simulink model "SVPWM"  (R2018b)
settings: Solver=FixedStepAuto  StartTime=0.0  StopTime=0.1  RelTol=1e-3
undefined symbols (not defined in the file): gcbh, Newton, Raphson, sps_rtmsupport
libraries: powerlib x60, powerlib_meascontrol x25, simulink x14, dspstat3 x1
(part 2 of 2)

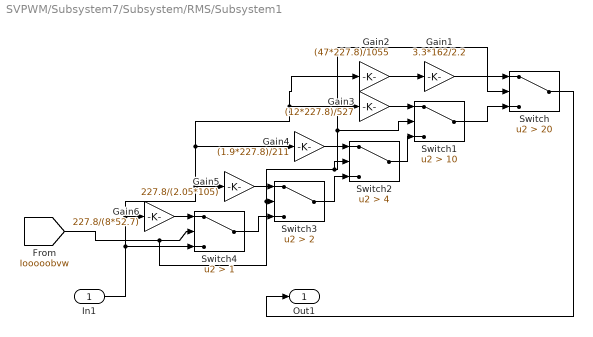
== system SVPWM/Subsystem7/Subsystem/RMS/Subsystem1 ==
  In1 : Inport
  Gain1 : Gain  Gain=3.3*162/2.2
  Gain2 : Gain  Gain=(47*227.8)/1055
  Gain3 : Gain  Gain=(12*227.8)/527
  Gain4 : Gain  Gain=(1.9*227.8)/211
  Gain5 : Gain  Gain=227.8/(2.05*105)
  Gain6 : Gain  Gain=227.8/(8*52.7)
  Switch : Switch  Criteria=u2 > Threshold  Threshold=20
  Switch1 : Switch  Criteria=u2 > Threshold  Threshold=10
  Switch2 : Switch  Criteria=u2 > Threshold  Threshold=4
  Switch3 : Switch  Criteria=u2 > Threshold  Threshold=2
  Switch4 : Switch  Criteria=u2 > Threshold  Threshold=1
  Out1 : Outport
  wires:
  Gain1/1 -> Switch/1
  Switch/1 -> Out1/1
  Gain6/1 -> Switch4/1
  Switch4/1 -> Switch3/3
  Switch2/1 -> Switch1/3
  Gain2/1 -> Gain1/1
  Gain5/1 -> Switch3/1
  Gain4/1 -> Switch2/1
  Switch3/1 -> Switch2/3
  Gain3/1 -> Switch1/1
  [Iooooobvw] -> Switch4/2, Switch3/2, Switch2/2, Switch1/2, Switch/2
  In1/1 -> Gain2/1, Gain3/1, Gain4/1, Gain5/1, Gain6/1, Switch4/3
  Switch1/1 -> Switch/3

== system SVPWM/Subsystem7/Subsystem/RMS/TrueRMS  ==
  In : Inport
  Enable : EnablePort
  Mean value : powerlib_meascontrol/Measurements/Mean  Freq=sps.Freq  Vinit=sps.Par_Init_TrueRMS  Ts=Ts
  Product : Product  SaturateOnIntegerOverflow=on  InputSameDT=on  OutDataTypeStr=Inherit: Same as first input
  Saturation to avoid negative sqrt : Saturate  UpperLimit=Inf  LowerLimit=0
  Sqrt : Sqrt  AlgorithmType=Newton-Raphson  SaturateOnIntegerOverflow=on
  RMS : Outport
  wires:
  Saturation to avoid negative sqrt/1 -> Sqrt/1
  Mean value/1 -> Saturation to avoid negative sqrt/1
  Product/1 -> Mean value/1
  In/1 -> Product/2, Product/1
  Sqrt/1 -> RMS/1

== system SVPWM/Subsystem7/Subsystem/Subsystem/Subsystem ==
  In1 : Inport
  In2 : Inport  Port=2
  Demux : Demux  Outputs=6
  Logical Operator : Logic  IconShape=distinctive  AllPortsSameDT=off  OutDataTypeStr=boolean
  Scope : Scope  NumInputPorts=2
  Switch : Switch  Criteria=u2 > Threshold
  Out1 : Outport
  wires:
  Demux/2 -> Scope/1, Switch/3
  Switch/1 -> Logical Operator/2
  [svpwm] -> Demux/1
  Logical Operator/1 -> Out1/1
  In1/1 -> Scope/2, Logical Operator/1
  In2/1 -> Switch/2

== system SVPWM/Subsystem7/Subsystem/Subsystem/Subsystem1 ==
  In1 : Inport
  In2 : Inport  Port=2
  Demux : Demux  Outputs=6
  Logical Operator : Logic  IconShape=distinctive  AllPortsSameDT=off  OutDataTypeStr=boolean
  SVPWM Generator (2-Level) : powerlib_meascontrol/Pulse & Signal Generators/SVPWM Generator (2-Level)  InputType=Internally generated  SwitchingPattern=Pattern #2  Fc=100  ParUref=[1 -60 50]  Ts=0
      settings: SourceProductName=Simscape Power Systems  SourceProductBaseCode=PS
  Scope : Scope  NumInputPorts=2
  Switch : Switch  Criteria=u2 > Threshold
  Out1 : Outport
  tag scope: svpwm=global
  wires:
  In2/1 -> Switch/2
  In1/1 -> Scope/2, Logical Operator/1
  Logical Operator/1 -> Out1/1
  SVPWM Generator (2-Level)/1 -> [svpwm], Demux/1
  Switch/1 -> Logical Operator/2
  Demux/1 -> Scope/1, Switch/1

== system SVPWM/Subsystem7/Subsystem1/RMS/RMS  ==
  In : Inport
  Enable : EnablePort
  Fourier1 : powerlib_meascontrol/Measurements/Fourier  Freq=sps.Freq  n=1  InInit=sps.Par_Init_RMS  Ts=Ts
      settings: SourceProductName=Simscape Power Systems
  Gain : Gain  Gain=1/sqrt(2)
  Terminator : Terminator
  RMS : Outport
  wires:
  Fourier1/1 -> Gain/1
  Fourier1/2 -> Terminator/1
  In/1 -> Fourier1/1
  Gain/1 -> RMS/1

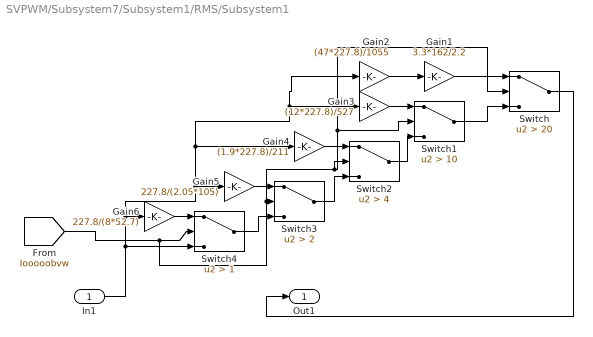
== system SVPWM/Subsystem7/Subsystem1/RMS/Subsystem1 ==
  In1 : Inport
  Gain1 : Gain  Gain=3.3*162/2.2
  Gain2 : Gain  Gain=(47*227.8)/1055
  Gain3 : Gain  Gain=(12*227.8)/527
  Gain4 : Gain  Gain=(1.9*227.8)/211
  Gain5 : Gain  Gain=227.8/(2.05*105)
  Gain6 : Gain  Gain=227.8/(8*52.7)
  Switch : Switch  Criteria=u2 > Threshold  Threshold=20
  Switch1 : Switch  Criteria=u2 > Threshold  Threshold=10
  Switch2 : Switch  Criteria=u2 > Threshold  Threshold=4
  Switch3 : Switch  Criteria=u2 > Threshold  Threshold=2
  Switch4 : Switch  Criteria=u2 > Threshold  Threshold=1
  Out1 : Outport
  wires:
  Gain1/1 -> Switch/1
  Switch/1 -> Out1/1
  Gain6/1 -> Switch4/1
  Switch4/1 -> Switch3/3
  Switch2/1 -> Switch1/3
  Gain2/1 -> Gain1/1
  Gain5/1 -> Switch3/1
  Gain4/1 -> Switch2/1
  Switch3/1 -> Switch2/3
  Gain3/1 -> Switch1/1
  [Iooooobvw] -> Switch4/2, Switch3/2, Switch2/2, Switch1/2, Switch/2
  In1/1 -> Gain2/1, Gain3/1, Gain4/1, Gain5/1, Gain6/1, Switch4/3
  Switch1/1 -> Switch/3

== system SVPWM/Subsystem7/Subsystem1/RMS/TrueRMS  ==
  In : Inport
  Enable : EnablePort
  Mean value : powerlib_meascontrol/Measurements/Mean  Freq=sps.Freq  Vinit=sps.Par_Init_TrueRMS  Ts=Ts
  Product : Product  SaturateOnIntegerOverflow=on  InputSameDT=on  OutDataTypeStr=Inherit: Same as first input
  Saturation to avoid negative sqrt : Saturate  UpperLimit=Inf  LowerLimit=0
  Sqrt : Sqrt  AlgorithmType=Newton-Raphson  SaturateOnIntegerOverflow=on
  RMS : Outport
  wires:
  Saturation to avoid negative sqrt/1 -> Sqrt/1
  Mean value/1 -> Saturation to avoid negative sqrt/1
  Product/1 -> Mean value/1
  In/1 -> Product/2, Product/1
  Sqrt/1 -> RMS/1

== system SVPWM/Subsystem7/Subsystem1/Subsystem7/Subsystem ==
  In1 : Inport
  In2 : Inport  Port=2
  Demux : Demux  Outputs=6
  Logical Operator : Logic  IconShape=distinctive  AllPortsSameDT=off  OutDataTypeStr=boolean
  Scope : Scope  NumInputPorts=2
  Switch : Switch  Criteria=u2 > Threshold
  Out1 : Outport
  wires:
  Demux/2 -> Scope/1, Switch/3
  Switch/1 -> Logical Operator/2
  [svpwm] -> Demux/1
  Logical Operator/1 -> Out1/1
  In1/1 -> Scope/2, Logical Operator/1
  In2/1 -> Switch/2

== system SVPWM/Subsystem7/Subsystem1/Subsystem7/Subsystem1 ==
  In1 : Inport
  In2 : Inport  Port=2
  Demux : Demux  Outputs=6
  Logical Operator : Logic  IconShape=distinctive  AllPortsSameDT=off  OutDataTypeStr=boolean
  Scope : Scope  NumInputPorts=2
  Switch : Switch  Criteria=u2 > Threshold
  Out1 : Outport
  wires:
  In2/1 -> Switch/2
  In1/1 -> Scope/2, Logical Operator/1
  Logical Operator/1 -> Out1/1
  [svpwm] -> Demux/1
  Switch/1 -> Logical Operator/2
  Demux/1 -> Scope/1, Switch/1

== system SVPWM/Subsystem7/Subsystem2/RMS/RMS  ==
  In : Inport
  Enable : EnablePort
  Fourier1 : powerlib_meascontrol/Measurements/Fourier  Freq=sps.Freq  n=1  InInit=sps.Par_Init_RMS  Ts=Ts
      settings: SourceProductName=Simscape Power Systems
  Gain : Gain  Gain=1/sqrt(2)
  Terminator : Terminator
  RMS : Outport
  wires:
  Fourier1/1 -> Gain/1
  Fourier1/2 -> Terminator/1
  In/1 -> Fourier1/1
  Gain/1 -> RMS/1

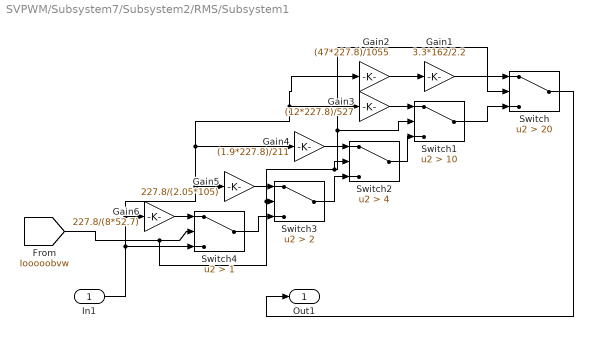
== system SVPWM/Subsystem7/Subsystem2/RMS/Subsystem1 ==
  In1 : Inport
  Gain1 : Gain  Gain=3.3*162/2.2
  Gain2 : Gain  Gain=(47*227.8)/1055
  Gain3 : Gain  Gain=(12*227.8)/527
  Gain4 : Gain  Gain=(1.9*227.8)/211
  Gain5 : Gain  Gain=227.8/(2.05*105)
  Gain6 : Gain  Gain=227.8/(8*52.7)
  Switch : Switch  Criteria=u2 > Threshold  Threshold=20
  Switch1 : Switch  Criteria=u2 > Threshold  Threshold=10
  Switch2 : Switch  Criteria=u2 > Threshold  Threshold=4
  Switch3 : Switch  Criteria=u2 > Threshold  Threshold=2
  Switch4 : Switch  Criteria=u2 > Threshold  Threshold=1
  Out1 : Outport
  wires:
  Gain1/1 -> Switch/1
  Switch/1 -> Out1/1
  Gain6/1 -> Switch4/1
  Switch4/1 -> Switch3/3
  Switch2/1 -> Switch1/3
  Gain2/1 -> Gain1/1
  Gain5/1 -> Switch3/1
  Gain4/1 -> Switch2/1
  Switch3/1 -> Switch2/3
  Gain3/1 -> Switch1/1
  [Iooooobvw] -> Switch4/2, Switch3/2, Switch2/2, Switch1/2, Switch/2
  In1/1 -> Gain2/1, Gain3/1, Gain4/1, Gain5/1, Gain6/1, Switch4/3
  Switch1/1 -> Switch/3

== system SVPWM/Subsystem7/Subsystem2/RMS/TrueRMS  ==
  In : Inport
  Enable : EnablePort
  Mean value : powerlib_meascontrol/Measurements/Mean  Freq=sps.Freq  Vinit=sps.Par_Init_TrueRMS  Ts=Ts
  Product : Product  SaturateOnIntegerOverflow=on  InputSameDT=on  OutDataTypeStr=Inherit: Same as first input
  Saturation to avoid negative sqrt : Saturate  UpperLimit=Inf  LowerLimit=0
  Sqrt : Sqrt  AlgorithmType=Newton-Raphson  SaturateOnIntegerOverflow=on
  RMS : Outport
  wires:
  Saturation to avoid negative sqrt/1 -> Sqrt/1
  Mean value/1 -> Saturation to avoid negative sqrt/1
  Product/1 -> Mean value/1
  In/1 -> Product/2, Product/1
  Sqrt/1 -> RMS/1

== system SVPWM/Subsystem7/Subsystem2/Subsystem/Subsystem ==
  In1 : Inport
  In2 : Inport  Port=2
  Demux : Demux  Outputs=6
  Logical Operator : Logic  IconShape=distinctive  AllPortsSameDT=off  OutDataTypeStr=boolean
  Scope : Scope  NumInputPorts=2
  Switch : Switch  Criteria=u2 > Threshold
  Out1 : Outport
  wires:
  Demux/2 -> Scope/1, Switch/3
  Switch/1 -> Logical Operator/2
  [svpwm] -> Demux/1
  Logical Operator/1 -> Out1/1
  In1/1 -> Scope/2, Logical Operator/1
  In2/1 -> Switch/2

== system SVPWM/Subsystem7/Subsystem2/Subsystem/Subsystem1 ==
  In1 : Inport
  In2 : Inport  Port=2
  Demux : Demux  Outputs=6
  Logical Operator : Logic  IconShape=distinctive  AllPortsSameDT=off  OutDataTypeStr=boolean
  Scope : Scope  NumInputPorts=2
  Switch : Switch  Criteria=u2 > Threshold
  Out1 : Outport
  wires:
  In2/1 -> Switch/2
  In1/1 -> Scope/2, Logical Operator/1
  Logical Operator/1 -> Out1/1
  [svpwm] -> Demux/1
  Switch/1 -> Logical Operator/2
  Demux/1 -> Scope/1, Switch/1

== system SVPWM/Subsystem7/Subsystem3/RMS/RMS  ==
  In : Inport
  Enable : EnablePort
  Fourier1 : powerlib_meascontrol/Measurements/Fourier  Freq=sps.Freq  n=1  InInit=sps.Par_Init_RMS  Ts=Ts
      settings: SourceProductName=Simscape Power Systems
  Gain : Gain  Gain=1/sqrt(2)
  Terminator : Terminator
  RMS : Outport
  wires:
  Fourier1/1 -> Gain/1
  Fourier1/2 -> Terminator/1
  In/1 -> Fourier1/1
  Gain/1 -> RMS/1

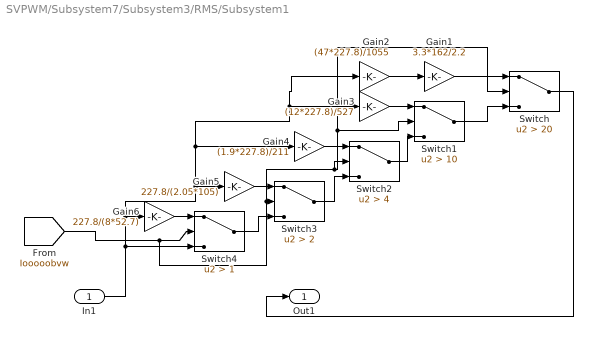
== system SVPWM/Subsystem7/Subsystem3/RMS/Subsystem1 ==
  In1 : Inport
  Gain1 : Gain  Gain=3.3*162/2.2
  Gain2 : Gain  Gain=(47*227.8)/1055
  Gain3 : Gain  Gain=(12*227.8)/527
  Gain4 : Gain  Gain=(1.9*227.8)/211
  Gain5 : Gain  Gain=227.8/(2.05*105)
  Gain6 : Gain  Gain=227.8/(8*52.7)
  Switch : Switch  Criteria=u2 > Threshold  Threshold=20
  Switch1 : Switch  Criteria=u2 > Threshold  Threshold=10
  Switch2 : Switch  Criteria=u2 > Threshold  Threshold=4
  Switch3 : Switch  Criteria=u2 > Threshold  Threshold=2
  Switch4 : Switch  Criteria=u2 > Threshold  Threshold=1
  Out1 : Outport
  wires:
  Gain1/1 -> Switch/1
  Switch/1 -> Out1/1
  Gain6/1 -> Switch4/1
  Switch4/1 -> Switch3/3
  Switch2/1 -> Switch1/3
  Gain2/1 -> Gain1/1
  Gain5/1 -> Switch3/1
  Gain4/1 -> Switch2/1
  Switch3/1 -> Switch2/3
  Gain3/1 -> Switch1/1
  [Iooooobvw] -> Switch4/2, Switch3/2, Switch2/2, Switch1/2, Switch/2
  In1/1 -> Gain2/1, Gain3/1, Gain4/1, Gain5/1, Gain6/1, Switch4/3
  Switch1/1 -> Switch/3

== system SVPWM/Subsystem7/Subsystem3/RMS/TrueRMS  ==
  In : Inport
  Enable : EnablePort
  Mean value : powerlib_meascontrol/Measurements/Mean  Freq=sps.Freq  Vinit=sps.Par_Init_TrueRMS  Ts=Ts
  Product : Product  SaturateOnIntegerOverflow=on  InputSameDT=on  OutDataTypeStr=Inherit: Same as first input
  Saturation to avoid negative sqrt : Saturate  UpperLimit=Inf  LowerLimit=0
  Sqrt : Sqrt  AlgorithmType=Newton-Raphson  SaturateOnIntegerOverflow=on
  RMS : Outport
  wires:
  Saturation to avoid negative sqrt/1 -> Sqrt/1
  Mean value/1 -> Saturation to avoid negative sqrt/1
  Product/1 -> Mean value/1
  In/1 -> Product/2, Product/1
  Sqrt/1 -> RMS/1

== system SVPWM/Subsystem7/Subsystem3/Subsystem/Subsystem ==
  In1 : Inport
  In2 : Inport  Port=2
  Demux : Demux  Outputs=6
  Logical Operator : Logic  IconShape=distinctive  AllPortsSameDT=off  OutDataTypeStr=boolean
  Scope : Scope  NumInputPorts=2
  Switch : Switch  Criteria=u2 > Threshold
  Out1 : Outport
  wires:
  Demux/2 -> Scope/1, Switch/3
  Switch/1 -> Logical Operator/2
  [svpwm] -> Demux/1
  Logical Operator/1 -> Out1/1
  In1/1 -> Scope/2, Logical Operator/1
  In2/1 -> Switch/2

== system SVPWM/Subsystem7/Subsystem3/Subsystem/Subsystem1 ==
  In1 : Inport
  In2 : Inport  Port=2
  Demux : Demux  Outputs=6
  Logical Operator : Logic  IconShape=distinctive  AllPortsSameDT=off  OutDataTypeStr=boolean
  Scope : Scope  NumInputPorts=2
  Switch : Switch  Criteria=u2 > Threshold
  Out1 : Outport
  wires:
  In2/1 -> Switch/2
  In1/1 -> Scope/2, Logical Operator/1
  Logical Operator/1 -> Out1/1
  [svpwm] -> Demux/1
  Switch/1 -> Logical Operator/2
  Demux/1 -> Scope/1, Switch/1

== system SVPWM/Subsystem7/Subsystem4/RMS/RMS  ==
  In : Inport
  Enable : EnablePort
  Fourier1 : powerlib_meascontrol/Measurements/Fourier  Freq=sps.Freq  n=1  InInit=sps.Par_Init_RMS  Ts=Ts
      settings: SourceProductName=Simscape Power Systems
  Gain : Gain  Gain=1/sqrt(2)
  Terminator : Terminator
  RMS : Outport
  wires:
  Fourier1/1 -> Gain/1
  Fourier1/2 -> Terminator/1
  In/1 -> Fourier1/1
  Gain/1 -> RMS/1

== system SVPWM/Subsystem7/Subsystem4/RMS/Subsystem1 ==
  In1 : Inport
  Gain1 : Gain  Gain=3.3*162/2.2
  Gain2 : Gain  Gain=(47*227.8)/1055
  Gain3 : Gain  Gain=(12*227.8)/527
  Gain4 : Gain  Gain=(1.9*227.8)/211
  Gain5 : Gain  Gain=227.8/(2.05*105)
  Gain6 : Gain  Gain=227.8/(8*52.7)
  Switch : Switch  Criteria=u2 > Threshold  Threshold=20
  Switch1 : Switch  Criteria=u2 > Threshold  Threshold=10
  Switch2 : Switch  Criteria=u2 > Threshold  Threshold=4
  Switch3 : Switch  Criteria=u2 > Threshold  Threshold=2
  Switch4 : Switch  Criteria=u2 > Threshold  Threshold=1
  Out1 : Outport
  wires:
  Gain1/1 -> Switch/1
  Switch/1 -> Out1/1
  Gain6/1 -> Switch4/1
  Switch4/1 -> Switch3/3
  Switch2/1 -> Switch1/3
  Gain2/1 -> Gain1/1
  Gain5/1 -> Switch3/1
  Gain4/1 -> Switch2/1
  Switch3/1 -> Switch2/3
  Gain3/1 -> Switch1/1
  [Iooooobvw] -> Switch4/2, Switch3/2, Switch2/2, Switch1/2, Switch/2
  In1/1 -> Gain2/1, Gain3/1, Gain4/1, Gain5/1, Gain6/1, Switch4/3
  Switch1/1 -> Switch/3

== system SVPWM/Subsystem7/Subsystem4/RMS/TrueRMS  ==
  In : Inport
  Enable : EnablePort
  Mean value : powerlib_meascontrol/Measurements/Mean  Freq=sps.Freq  Vinit=sps.Par_Init_TrueRMS  Ts=Ts
  Product : Product  SaturateOnIntegerOverflow=on  InputSameDT=on  OutDataTypeStr=Inherit: Same as first input
  Saturation to avoid negative sqrt : Saturate  UpperLimit=Inf  LowerLimit=0
  Sqrt : Sqrt  AlgorithmType=Newton-Raphson  SaturateOnIntegerOverflow=on
  RMS : Outport
  wires:
  Saturation to avoid negative sqrt/1 -> Sqrt/1
  Mean value/1 -> Saturation to avoid negative sqrt/1
  Product/1 -> Mean value/1
  In/1 -> Product/2, Product/1
  Sqrt/1 -> RMS/1

== system SVPWM/Subsystem7/Subsystem4/Subsystem/Subsystem ==
  In1 : Inport
  In2 : Inport  Port=2
  Demux : Demux  Outputs=6
  Logical Operator : Logic  IconShape=distinctive  AllPortsSameDT=off  OutDataTypeStr=boolean
  Scope : Scope  NumInputPorts=2
  Switch : Switch  Criteria=u2 > Threshold
  Out1 : Outport
  wires:
  Demux/2 -> Scope/1, Switch/3
  Switch/1 -> Logical Operator/2
  [svpwm] -> Demux/1
  Logical Operator/1 -> Out1/1
  In1/1 -> Scope/2, Logical Operator/1
  In2/1 -> Switch/2

== system SVPWM/Subsystem7/Subsystem4/Subsystem/Subsystem1 ==
  In1 : Inport
  In2 : Inport  Port=2
  Demux : Demux  Outputs=6
  Logical Operator : Logic  IconShape=distinctive  AllPortsSameDT=off  OutDataTypeStr=boolean
  Scope : Scope  NumInputPorts=2
  Switch : Switch  Criteria=u2 > Threshold
  Out1 : Outport
  wires:
  In2/1 -> Switch/2
  In1/1 -> Scope/2, Logical Operator/1
  Logical Operator/1 -> Out1/1
  [svpwm] -> Demux/1
  Switch/1 -> Logical Operator/2
  Demux/1 -> Scope/1, Switch/1

== system SVPWM/Subsystem7/Subsystem5/RMS/RMS  ==
  In : Inport
  Enable : EnablePort
  Fourier1 : powerlib_meascontrol/Measurements/Fourier  Freq=sps.Freq  n=1  InInit=sps.Par_Init_RMS  Ts=Ts
      settings: SourceProductName=Simscape Power Systems
  Gain : Gain  Gain=1/sqrt(2)
  Terminator : Terminator
  RMS : Outport
  wires:
  Fourier1/1 -> Gain/1
  Fourier1/2 -> Terminator/1
  In/1 -> Fourier1/1
  Gain/1 -> RMS/1

== system SVPWM/Subsystem7/Subsystem5/RMS/Subsystem1 ==
  In1 : Inport
  Gain1 : Gain  Gain=3.3*162/2.2
  Gain2 : Gain  Gain=(47*227.8)/1055
  Gain3 : Gain  Gain=(12*227.8)/527
  Gain4 : Gain  Gain=(1.9*227.8)/211
  Gain5 : Gain  Gain=227.8/(2.05*105)
  Gain6 : Gain  Gain=227.8/(8*52.7)
  Switch : Switch  Criteria=u2 > Threshold  Threshold=20
  Switch1 : Switch  Criteria=u2 > Threshold  Threshold=10
  Switch2 : Switch  Criteria=u2 > Threshold  Threshold=4
  Switch3 : Switch  Criteria=u2 > Threshold  Threshold=2
  Switch4 : Switch  Criteria=u2 > Threshold  Threshold=1
  Out1 : Outport
  wires:
  Gain1/1 -> Switch/1
  Switch/1 -> Out1/1
  Gain6/1 -> Switch4/1
  Switch4/1 -> Switch3/3
  Switch2/1 -> Switch1/3
  Gain2/1 -> Gain1/1
  Gain5/1 -> Switch3/1
  Gain4/1 -> Switch2/1
  Switch3/1 -> Switch2/3
  Gain3/1 -> Switch1/1
  [Iooooobvw] -> Switch4/2, Switch3/2, Switch2/2, Switch1/2, Switch/2
  In1/1 -> Gain2/1, Gain3/1, Gain4/1, Gain5/1, Gain6/1, Switch4/3
  Switch1/1 -> Switch/3

== system SVPWM/Subsystem7/Subsystem5/RMS/TrueRMS  ==
  In : Inport
  Enable : EnablePort
  Mean value : powerlib_meascontrol/Measurements/Mean  Freq=sps.Freq  Vinit=sps.Par_Init_TrueRMS  Ts=Ts
  Product : Product  SaturateOnIntegerOverflow=on  InputSameDT=on  OutDataTypeStr=Inherit: Same as first input
  Saturation to avoid negative sqrt : Saturate  UpperLimit=Inf  LowerLimit=0
  Sqrt : Sqrt  AlgorithmType=Newton-Raphson  SaturateOnIntegerOverflow=on
  RMS : Outport
  wires:
  Saturation to avoid negative sqrt/1 -> Sqrt/1
  Mean value/1 -> Saturation to avoid negative sqrt/1
  Product/1 -> Mean value/1
  In/1 -> Product/2, Product/1
  Sqrt/1 -> RMS/1

== system SVPWM/Subsystem7/Subsystem5/Subsystem/Subsystem ==
  In1 : Inport
  In2 : Inport  Port=2
  Demux : Demux  Outputs=6
  Logical Operator : Logic  IconShape=distinctive  AllPortsSameDT=off  OutDataTypeStr=boolean
  Scope : Scope  NumInputPorts=2
  Switch : Switch  Criteria=u2 > Threshold
  Out1 : Outport
  wires:
  Demux/2 -> Scope/1, Switch/3
  Switch/1 -> Logical Operator/2
  [svpwm] -> Demux/1
  Logical Operator/1 -> Out1/1
  In1/1 -> Scope/2, Logical Operator/1
  In2/1 -> Switch/2

== system SVPWM/Subsystem7/Subsystem5/Subsystem/Subsystem1 ==
  In1 : Inport
  In2 : Inport  Port=2
  Demux : Demux  Outputs=6
  Logical Operator : Logic  IconShape=distinctive  AllPortsSameDT=off  OutDataTypeStr=boolean
  Scope : Scope  NumInputPorts=2
  Switch : Switch  Criteria=u2 > Threshold
  Out1 : Outport
  wires:
  In2/1 -> Switch/2
  In1/1 -> Scope/2, Logical Operator/1
  Logical Operator/1 -> Out1/1
  [svpwm] -> Demux/1
  Switch/1 -> Logical Operator/2
  Demux/1 -> Scope/1, Switch/1

== system SVPWM/Subsystem7/Subsystem6/RMS/RMS  ==
  In : Inport
  Enable : EnablePort
  Fourier1 : powerlib_meascontrol/Measurements/Fourier  Freq=sps.Freq  n=1  InInit=sps.Par_Init_RMS  Ts=Ts
      settings: SourceProductName=Simscape Power Systems
  Gain : Gain  Gain=1/sqrt(2)
  Terminator : Terminator
  RMS : Outport
  wires:
  Fourier1/1 -> Gain/1
  Fourier1/2 -> Terminator/1
  In/1 -> Fourier1/1
  Gain/1 -> RMS/1

== system SVPWM/Subsystem7/Subsystem6/RMS/Subsystem1 ==
  In1 : Inport
  Gain1 : Gain  Gain=3.3*162/2.2
  Gain2 : Gain  Gain=(47*227.8)/1055
  Gain3 : Gain  Gain=(12*227.8)/527
  Gain4 : Gain  Gain=(1.9*227.8)/211
  Gain5 : Gain  Gain=227.8/(2.05*105)
  Gain6 : Gain  Gain=227.8/(8*52.7)
  Switch : Switch  Criteria=u2 > Threshold  Threshold=20
  Switch1 : Switch  Criteria=u2 > Threshold  Threshold=10
  Switch2 : Switch  Criteria=u2 > Threshold  Threshold=4
  Switch3 : Switch  Criteria=u2 > Threshold  Threshold=2
  Switch4 : Switch  Criteria=u2 > Threshold  Threshold=1
  Out1 : Outport
  wires:
  Gain1/1 -> Switch/1
  Switch/1 -> Out1/1
  Gain6/1 -> Switch4/1
  Switch4/1 -> Switch3/3
  Switch2/1 -> Switch1/3
  Gain2/1 -> Gain1/1
  Gain5/1 -> Switch3/1
  Gain4/1 -> Switch2/1
  Switch3/1 -> Switch2/3
  Gain3/1 -> Switch1/1
  [Iooooobvw] -> Switch4/2, Switch3/2, Switch2/2, Switch1/2, Switch/2
  In1/1 -> Gain2/1, Gain3/1, Gain4/1, Gain5/1, Gain6/1, Switch4/3
  Switch1/1 -> Switch/3

== system SVPWM/Subsystem7/Subsystem6/RMS/TrueRMS  ==
  In : Inport
  Enable : EnablePort
  Mean value : powerlib_meascontrol/Measurements/Mean  Freq=sps.Freq  Vinit=sps.Par_Init_TrueRMS  Ts=Ts
  Product : Product  SaturateOnIntegerOverflow=on  InputSameDT=on  OutDataTypeStr=Inherit: Same as first input
  Saturation to avoid negative sqrt : Saturate  UpperLimit=Inf  LowerLimit=0
  Sqrt : Sqrt  AlgorithmType=Newton-Raphson  SaturateOnIntegerOverflow=on
  RMS : Outport
  wires:
  Saturation to avoid negative sqrt/1 -> Sqrt/1
  Mean value/1 -> Saturation to avoid negative sqrt/1
  Product/1 -> Mean value/1
  In/1 -> Product/2, Product/1
  Sqrt/1 -> RMS/1

== system SVPWM/Subsystem7/Subsystem6/Subsystem/Subsystem ==
  In1 : Inport
  In2 : Inport  Port=2
  Demux : Demux  Outputs=6
  Logical Operator : Logic  IconShape=distinctive  AllPortsSameDT=off  OutDataTypeStr=boolean
  Scope : Scope  NumInputPorts=2
  Switch : Switch  Criteria=u2 > Threshold
  Out1 : Outport
  wires:
  Demux/2 -> Scope/1, Switch/3
  Switch/1 -> Logical Operator/2
  [svpwm] -> Demux/1
  Logical Operator/1 -> Out1/1
  In1/1 -> Scope/2, Logical Operator/1
  In2/1 -> Switch/2

== system SVPWM/Subsystem7/Subsystem6/Subsystem/Subsystem1 ==
  In1 : Inport
  In2 : Inport  Port=2
  Demux : Demux  Outputs=6
  Logical Operator : Logic  IconShape=distinctive  AllPortsSameDT=off  OutDataTypeStr=boolean
  Scope : Scope  NumInputPorts=2
  Switch : Switch  Criteria=u2 > Threshold
  Out1 : Outport
  wires:
  In2/1 -> Switch/2
  In1/1 -> Scope/2, Logical Operator/1
  Logical Operator/1 -> Out1/1
  [svpwm] -> Demux/1
  Switch/1 -> Logical Operator/2
  Demux/1 -> Scope/1, Switch/1
